simulink model "TwoMasssystemRigid_v2"  (Simulink 7.0)
settings: Solver=ode4  StartTime=0.0  StopTime=tstop  FixedStep=h_v2  RelTol=1e-8
values from neighbouring files (symbols this model uses):
  f = 10    [main.m]
  Fmax = 100    [main.m]
  k = 1e+4    (= 10000)    [main.m]
  m1 = 0.1    [main.m]
  m2 = 0.2    [main.m]
  y1_0 = y2_0    (= 0)    [main.m]
  y1p_0 = y2p_0    (= 0)    [main.m]
  y2_0 = 0    [main.m]
  y2p_0 = 0    [main.m]
settings Model: Creator=adminus  LastModifiedBy=adminus

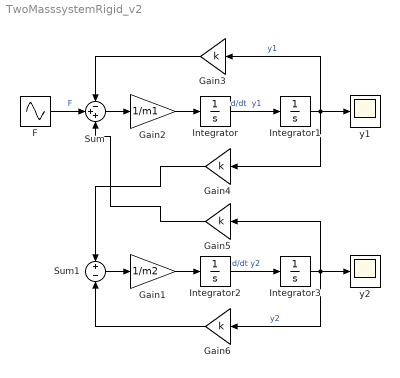
== system TwoMasssystemRigid_v2 ==
  F : Sin  Amplitude=Fmax  Frequency=2*pi*f  SampleTime=0
  Gain1 : Gain  Gain=1/m2  ParameterDataType=sfix(16)  ParameterScaling=2^0  OutDataType=sfix(16)  OutScaling=2^0
  Gain2 : Gain  Gain=1/m1  ParameterDataType=sfix(16)  ParameterScaling=2^0  OutDataType=sfix(16)  OutScaling=2^0
  Gain{3..6} (4 alike) : Gain  Orientation=left  Gain=k  ParameterDataType=sfix(16)  ParameterScaling=2^0  OutDataType=sfix(16)  OutScaling=2^0
  Integrator : Integrator  InitialCondition=y1p_0
  Integrator1 : Integrator  InitialCondition=y1_0
  Integrator2 : Integrator  InitialCondition=y2p_0
  Integrator3 : Integrator  InitialCondition=y2_0
  Sum : Sum  Inputs=-++  OutDataType=sfix(16)  OutScaling=2^0
  Sum1 : Sum  Inputs=+|-  OutDataType=sfix(16)  OutScaling=2^0
  y1 : Scope
      settings: TimeRange=0.3  YMin=0  YMax=3.25  SaveName=ScopeData_v2_y1
  y2 : Scope
  wires:
  Integrator/1 -> Integrator1/1  "d/dt  y1"
  Integrator1/1 -> y1/1, Gain3/1, Gain4/1  "y1"
  Integrator2/1 -> Integrator3/1  "d/dt y2"
  Integrator3/1 -> y2/1, Gain6/1, Gain5/1  "y2"
  Gain2/1 -> Integrator/1
  Gain1/1 -> Integrator2/1
  F/1 -> Sum/2  "F"
  Sum/1 -> Gain2/1
  Gain3/1 -> Sum/1
  Gain4/1 -> Sum1/1
  Gain5/1 -> Sum/3
  Sum1/1 -> Gain1/1
  Gain6/1 -> Sum1/2
